simulink model "bio_matfunc_dumpModeSwitch"  (R2017b)
settings: Solver=VariableStepAuto  StartTime=0.0  StopTime=10.0  RelTol=1e-3
settings Model: Creator=ktrinh  LastModifiedBy=ktrinh

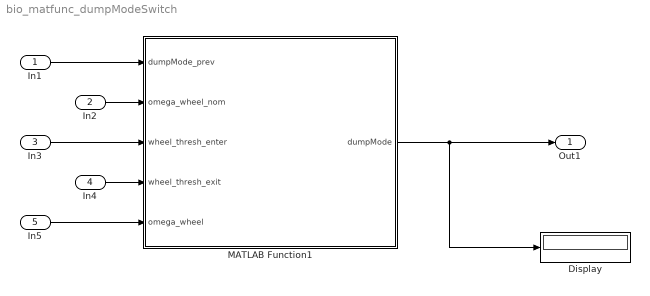
== system bio_matfunc_dumpModeSwitch ==
  In1 : Inport  OutDataTypeStr=double  PortDimensions=1
  In2 : Inport  Port=2  OutDataTypeStr=double  PortDimensions=1
  In3 : Inport  Port=3  OutDataTypeStr=double  PortDimensions=1
  In4 : Inport  Port=4  OutDataTypeStr=double  PortDimensions=1
  In5 : Inport  Port=5  OutDataTypeStr=double  PortDimensions=3
  Display : Display
  MATLAB Function1 : MATLAB Function  TreatAsAtomicUnit=on
  Out1 : Outport
  wires:
  MATLAB Function1/1(dumpMode) -> Display/1, Out1/1
  In1/1 -> MATLAB Function1/1(dumpMode_prev)
  In2/1 -> MATLAB Function1/2(omega_wheel_nom)
  In3/1 -> MATLAB Function1/3(wheel_thresh_enter)
  In4/1 -> MATLAB Function1/4(wheel_thresh_exit)
  In5/1 -> MATLAB Function1/5(omega_wheel)

== matlab function bio_matfunc_dumpModeSwitch/MATLAB Function1 ==
  data: dumpMode_prev input; omega_wheel_nom input; wheel_thresh_enter input; wheel_thresh_exit input; dumpMode output; omega_wheel input
function dumpMode = dumpModeSwitch(dumpMode_prev,omega_wheel_nom,wheel_thresh_enter,wheel_thresh_exit,omega_wheel)
%#codegen

if dumpMode_prev == 0
    if abs(omega_wheel(1) - omega_wheel_nom) > wheel_thresh_enter || abs(omega_wheel(2) - omega_wheel_nom) > wheel_thresh_enter || abs(omega_wheel(3) - omega_wheel_nom) > wheel_thresh_enter
        dumpMode = 1;
    else
        dumpMode = 0;
    end
elseif dumpMode_prev == 1
    if abs(omega_wheel(1) - omega_wheel_nom) < wheel_thresh_exit && abs(omega_wheel(2) - omega_wheel_nom) < wheel_thresh_exit && abs(omega_wheel(3) - omega_wheel_nom) < wheel_thresh_exit
        dumpMode = 0;
    else
        dumpMode = 1;
    end
else
    dumpMode = 0;
end
